simulink model "demodApproach4"  (Simulink 8.6)
settings: Solver=VariableStepAuto  SolverMode=SingleTasking  StartTime=0.0  StopTime=0.0075  MaxStep=0.01/2400  RelTol=1e-3
undefined symbols (not defined in the file): DiscIntNeverNeededParam
libraries: dsparch4 x2
settings Model: Creator=Aravind S  LastModifiedBy=Pranay
settings DataIOCC: LimitDataPoints=off  SaveFormat=Dataset  SignalLoggingSaveFormat=Dataset  ReturnWorkspaceOutputs=on
settings OptimizationCC: ExpressionDepthLimit=128
settings DebuggingCC: UnderspecifiedInitializationDetection=Simplified  MergeDetectMultiDrivingBlocksExec=error  SolverPrmCheckMsg=none  FcnCallInpInsideContextMsg=EnableAllAsError  AllowSymbolicDim=on  StateNameClashWarn=none  SFUnexpectedBacktrackingDiag=error  SFNoUnconditionalDefaultTransitionDiag=error
settings HardwareCC: ProdBitPerPointer=64  ProdLargestAtomicFloat=Float  ProdIntDivRoundTo=Zero  ProdEndianess=LittleEndian  ProdWordSize=64  ProdHWDeviceType=Intel->x86-64 (Windows64)
settings ModelReferenceCC: PropagateSignalLabelsOutOfModel=on
settings SFSimCC: SimUseLocalCustomCode=on
settings RTWCC: RTWUseLocalCustomCode=on
settings GRTTargetCC: TargetLangStandard=C99 (ISO)  GeneratePreprocessorConditionals=Use local settings  CombineOutputUpdateFcns=on  GRTInterface=off
settings ConfigComp: CovMetricSettings=dwe  CovHtmlReporting=off  CovSaveCumulativeToWorkspaceVar=off  CovSaveSingleToWorkspaceVar=off  CovExternalEMLEnable=on

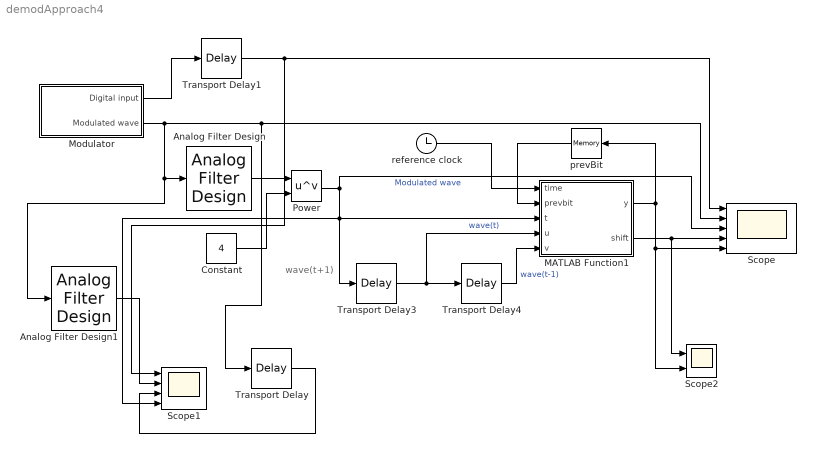
== system demodApproach4 ==
  note: wave(t+1)
  Analog Filter Design : dsparch4/Analog Filter Design  method=Bessel  filttype=Lowpass  N=15  Wlo=2*pi*1800  Whi=2*pi*1600  Rp=.01  Rs=60
  Analog Filter Design1 : dsparch4/Analog Filter Design  method=Bessel  filttype=Lowpass  N=15  Wlo=2*pi*1800  Whi=80  Rp=6  Rs=40
  Constant : Constant  Value=4
  MATLAB Function1 : MATLAB Function  TreatAsAtomicUnit=on
  Modulator : Subsystem
  Power : Math  Operator=pow  SaturateOnIntegerOverflow=on
  Scope : Scope  NumInputPorts=5
  Scope1 : Scope  NumInputPorts=4
  Scope2 : Scope  NumInputPorts=2
  Transport Delay : TransportDelay  DelayTime=1.0e-3
  Transport Delay1 : TransportDelay  DelayTime=1.0e-3
  Transport Delay3 : TransportDelay  DelayTime=0.05/2400
  Transport Delay4 : TransportDelay  DelayTime=0.05/2400
  prevBit : Memory
  reference clock : Clock
  wires:
  prevBit/1 -> MATLAB Function1/2(prevbit)
  reference clock/1 -> MATLAB Function1/1(time)
  Transport Delay4/1 -> MATLAB Function1/5(v)  "wave(t-1)"
  Analog Filter Design/1 -> Power/1
  Transport Delay3/1 -> MATLAB Function1/4(u), Transport Delay4/1  "wave(t)"
  Constant/1 -> Power/2
  MATLAB Function1/1(y) -> Scope/5, Scope2/2, prevBit/1
  Power/1 -> Scope/3, Scope1/4, Transport Delay3/1, MATLAB Function1/3(t)  "Modulated wave"
  Modulator/1(Digital input) -> Transport Delay1/1
  Modulator/2(Modulated wave) -> Analog Filter Design1/1, Analog Filter Design/1, Transport Delay/1, Scope/2
  Transport Delay1/1 -> Scope1/1, Scope/1
  MATLAB Function1/2(shift) -> Scope2/1, Scope/4
  Analog Filter Design1/1 -> Scope1/2
  Transport Delay/1 -> Scope1/3

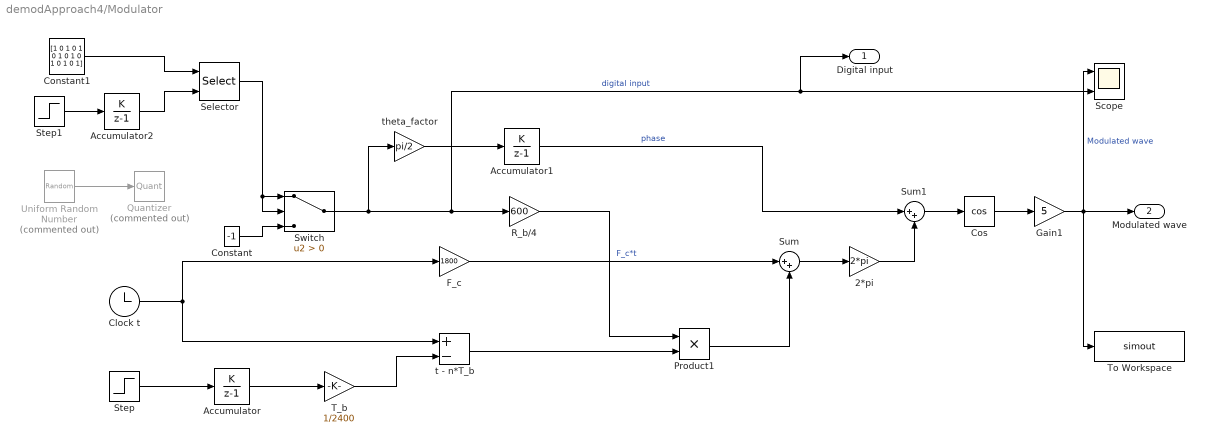
== system demodApproach4/Modulator ==
  2*pi : Gain  Gain=2*pi
  Accumulator : DiscreteIntegrator  IntegratorMethod=Accumulation: Forward Euler  InitialConditionSetting=State (most efficient)  SampleTime=-1  ICPrevOutput=DiscIntNeverNeededParam  ICPrevScaledInput=DiscIntNeverNeededParam
  Accumulator1 : DiscreteIntegrator  IntegratorMethod=Accumulation: Forward Euler  gainval=1  InitialConditionSetting=State (most efficient)  SampleTime=-1  ICPrevOutput=DiscIntNeverNeededParam  ICPrevScaledInput=DiscIntNeverNeededParam
  Accumulator2 : DiscreteIntegrator  IntegratorMethod=Accumulation: Forward Euler  gainval=1  InitialConditionSetting=State (most efficient)  SampleTime=-1  LimitOutput=on  UpperSaturationLimit=14  ICPrevOutput=DiscIntNeverNeededParam  ICPrevScaledInput=DiscIntNeverNeededParam
  Clock t : Clock
  Constant : Constant  Value=-1
  Constant1 : Constant  Value=[1 0 1 0 1 0 1 0 1 0 1 0 1 0 1]  SampleTime=0.1
  Cos : Trigonometry  Operator=cos
  F_c : Gain  Gain=1800
  Gain1 : Gain  Gain=5
  Product1 : Product
  Quantizer : Quantizer  Commented=on  QuantizationInterval=1
  R_b/4 : Gain  Gain=600
  Scope : Scope  NumInputPorts=2
  Selector : Selector  IndexMode=Zero-based  InputPortWidth=15  IndexOptions=Index vector (port)  Indices=1  OutputSizes=1
  Step : Step  Time=0  SampleTime=0
  Step1 : Step  Time=0  SampleTime=1/2400
  Sum : Sum  Inputs=|++
  Sum1 : Sum  Inputs=|++
  Switch : Switch  Criteria=u2 > Threshold
  T_b : Gain  Gain=1/2400
  To Workspace : ToWorkspace  VariableName=simout  SampleTime=-1
  Uniform Random Number : UniformRandomNumber  Commented=on  Minimum=0  Seed=5  SampleTime=1/2400
  t - n*T_b : Sum  Inputs=+-
  theta_factor : Gain  Gain=pi/2
  Digital input : Outport
  Modulated wave : Outport  Port=2
  wires:
  theta_factor/1 -> Accumulator1/1
  Sum/1 -> 2*pi/1
  Accumulator/1 -> T_b/1
  Clock t/1 -> t - n*T_b/1, F_c/1
  2*pi/1 -> Sum1/2
  Product1/1 -> Sum/2
  Cos/1 -> Gain1/1
  Gain1/1 -> Modulated wave/1, To Workspace/1, Scope/1  "Modulated wave"
  t - n*T_b/1 -> Product1/2
  R_b/4/1 -> Product1/1
  T_b/1 -> t - n*T_b/2
  F_c/1 -> Sum/1  "F_c*t"
  Switch/1 -> theta_factor/1, Digital input/1, Scope/2, R_b/4/1  "digital input"
  Uniform Random Number/1 -> Quantizer/1
  Step/1 -> Accumulator/1
  Accumulator1/1 -> Sum1/1  "phase"
  Constant/1 -> Switch/3
  Constant1/1 -> Selector/1
  Step1/1 -> Accumulator2/1
  Accumulator2/1 -> Selector/2
  Sum1/1 -> Cos/1
  Selector/1 -> Switch/2, Switch/1

== matlab function MATLAB Function1 ==
  data: time input double; prevbit input int8; t input double; u input double; y output double; v input double; shift output double
function [y, shift]  = fcn(time, prevbit, t, u, v)

%for finding local maximas
fdiff = t - u;
sdiff = u - v;

%for finding the first bit
if (prevbit == 0)
    if (u > 0.4 && time < 1.2e-3)
        k = -1;
    elseif (time > 1.2e-3)
        k = 1;
    else
        k = prevbit;
    end
    shift = 0;

%last clause in if is to handle edge cases where there might be extremely
%small local maximas less than 10e-6
elseif (fdiff < 0 && sdiff > 0 && u < 2 && max(abs(fdiff), abs(sdiff)) > 1e-5 && time > 1.3e-3)
    k = transition(prevbit);
    shift = 1;
else
    k = prevbit;
    shift = 0;
end

y = k;

function nextbit = transition(prevbit)
    if (prevbit == 0)
        nextbit = prevbit;
    elseif (prevbit < 0)
        nextbit = 1;
    else
        nextbit = -1;
    end
